simulink model "EE684_Project"  (R2023b)
settings: Solver=ode23t  StartTime=0.0  StopTime=1  RelTol=1e-3
undefined symbols (not defined in the file): acSupply, acSupplyController, bms, bmsController, boostController, connectedLoad, dcVoltage, Ion, Lithium, maxSoC, maxVdc, minIrrad, minSoC, minVdc, olTime, sensor, solarPanel, solarPlant
libraries: fl_lib x25, nesl_utility x23, ee_lib x12, spsSeriesRLCBranchLib x8, simulink x6, eePwmGenerator x4, spsIGBTDiodeLib x4, simulink_extras x2, spsCurrentMeasurementLib x2, spsMosfetLib x2, slpidlib x2, spsVoltageMeasurementLib x2
(part 2 of 2)

== system EE684_Project/AC System/AC Supply Controller ==
  note: Voltage Control
  note: Current control
  Modulating Signal : Subsystem
  Sine Wave1 : Sin  Amplitude=acSupply.supplyVoltage*1.414  Frequency=acSupply.frequency*2*pi  SampleTime=1/(30*2*pi*acSupply.frequency)
  Sum5 : Sum  Inputs=|+-
  Sum8 : Sum  Inputs=|+-
  Transfer Fcn1 : TransferFcn  Denominator=[1e-4 1]
  Voltage control2 : Subsystem
  d-axis current control2 : Subsystem
  act : Outport  VectorParamsAs1DForOutWhenUnconnected=off
  wires:
  Modulating Signal/1(m1) -> act/1
  d-axis current control2/1(u) -> Modulating Signal/1(Vmod)
  [Vo] -> Modulating Signal/2(Vdc)
  Sum8/1 -> Voltage control2/1(e)
  [Vs] -> Sum8/2
  [Iac] -> Sum5/2
  Sum5/1 -> d-axis current control2/1(e)
  Sine Wave1/1 -> Transfer Fcn1/1
  Voltage control2/1(u) -> Sum5/1
  Transfer Fcn1/1 -> Sum8/1

== system EE684_Project/AC System/Complex Load ==
  AC Voltage Sensor1 : Subsystem
      mask Display: disp('v')
  DC Current Sensor : Subsystem
      mask Display: disp('i')
  Inductor : ee_lib/Passive/Inductor  Commented=on  l=0 H  enable_L_tol=0  L_tol=5  tol_distribution=1  nSigma=4  r=0 Ohm  g=1e-9 1/Ohm  enable_operating_limits=0  operating_limit_action=2  max_working_current=1 A  power_rating=1 W  enable_faults=ee.enum.enable.no  fault_action=simscape.enum.assert.action.none  lambdaPercent=50  k_faulted=0.9999  turnsShort=0  openCct=0  groundShort=0  groundShortG=0 1/Ohm  tau_fault=1e-3 s  fault_trigger=ee.enum.faults.faultTrigger.temporal  t_fault=1 s  max_permissible_voltage=100 V  n_fail_on_voltage=1  max_permissible_current=1 A  t_fail_on_current=1 s  i_L_specify=off  i_L_priority=High  i_L=0 A  i_L_nominal_specify=off  i_L_nominal_unit=A  i_L_nominal_value=1
  Load Calculation : Subsystem
  Load Resistance : fl_lib/Electrical/Electrical Elements/Variable Resistor  Rmin=0 Ohm  thermalEnable=false  thermal_mass=1 J/K  i_specify=off  i_priority=None  i=5 A  i_nominal_specify=off  i_nominal_unit=A  i_nominal_value=1  v_specify=off  v_priority=None  v=0 V  v_nominal_specify=off  v_nominal_unit=V  v_nominal_value=1  T_specify=off  T_priority=None  T=300 K  T_nominal_specify=off  T_nominal_unit=K  T_nominal_value=1
  Variable Inductor : ee_lib/Passive/Variable Inductor  prm=1  Lmin=1e-6 H  g=1e-9 1/Ohm  i0=0 A  phi0=0 Wb
      settings: InternalSimscapePortConfiguration="{\"Bottom\":[],\"Left\":[{\"id\":\"L\",\"label\":\"L\",\"type\":\"input\"},{\"id\":\"p\",\"label\":\"+\",\"type\":\"foundation.electrical.electrical\"}],\"Right\":[{\"id\":\"n\",\"label\":\"-\",\"type\":\"foundation.electrical.electrical\"}],\"Top\":[]}"
  P : PMIOPort  Side=Left
  N : PMIOPort  Port=2  Side=Left
  connections:
  AC Voltage Sensor1/LConn1 -- N/RConn1 -- Variable Inductor/RConn1
  Load Resistance/LConn2 -- DC Current Sensor/LConn1
  DC Current Sensor/RConn1 -- P/RConn1 -- AC Voltage Sensor1/RConn1
  Variable Inductor/LConn2 -- Load Resistance/RConn1
  Load Calculation/RConn1 -- Load Resistance/LConn1
  Load Calculation/RConn2 -- Variable Inductor/LConn1

== system EE684_Project/AC System/Load Flag ==
  Data Type Conversion1 : DataTypeConversion  SaturateOnIntegerOverflow=off  RndMeth=Floor
  NOT : Logic  Operator=NOT  IconShape=distinctive  AllPortsSameDT=off  OutDataTypeStr=boolean
  OR : Logic  Operator=OR  IconShape=distinctive  AllPortsSameDT=off  OutDataTypeStr=boolean
  Simulink-PS Converter2 : nesl_utility/Simulink-PS Converter  PhysicalDomain=network_engine_domain  SubClassName=ps_input  LeftPortType=input  RightPortType=output  PseudoPeriodic=off  Frequencies=[]  NoiseDistribution=none  NoiseParameters=[]  Unit=1  AffineConversion=off  FilteringAndDerivatives=provide  SimscapeFilterOrder=1  InputFilterTimeConstant=0.001  UdotUserProvided=0
  CB : PMIOPort  Side=Right
  wires:
  [loadShutDown] -> OR/1
  Data Type Conversion1/1 -> Simulink-PS Converter2/1
  [ShutDown] -> OR/2  "System Status"
  OR/1 -> NOT/1
  NOT/1 -> Data Type Conversion1/1
  connections:
  Simulink-PS Converter2/RConn1 -- CB/RConn1

== system EE684_Project/AC System/Single Phase Inverter ==
  DC Current Sensor : Subsystem
      mask Display: disp('i')
  Power Circuit : Subsystem  Variant=on  VariantControl=Variant1
  + : PMIOPort  Side=Left
  P : PMIOPort  Port=2  Side=Right
  N : PMIOPort  Port=3  Side=Right
  - : PMIOPort  Port=4  Side=Left
  wires:
  [acMod] -> Power Circuit/1(m)
  [ShutDown] -> Power Circuit/2(TripSig)
  connections:
  +/RConn1 -- Power Circuit/LConn1
  -/RConn1 -- Power Circuit/LConn2
  P/RConn1 -- DC Current Sensor/LConn1
  N/RConn1 -- Power Circuit/RConn2
  DC Current Sensor/RConn1 -- Power Circuit/RConn1

== system EE684_Project/BMS/DC Battery Current Sensor1 ==
  Current Sensor : fl_lib/Electrical/Electrical Sensors/Current Sensor
  PS-Simulink Converter : nesl_utility/PS-Simulink Converter  PhysicalDomain=network_engine_domain  SubClassName=ps_output  LeftPortType=input  RightPortType=output  PseudoPeriodic=off  Frequencies=[]  VectorFormat=1-D array  Unit=1  AffineConversion=off
  Sensor dynamics : TransferFcn  Numerator=1  Denominator=[1/sensor.samplingFreq 1]
  - : PMIOPort  Side=Left
  + : PMIOPort  Port=2  Side=Right
  tag scope: Ibattery=global
  wires:
  PS-Simulink Converter/1 -> Sensor dynamics/1
  Sensor dynamics/1 -> [Ibattery]
  connections:
  Current Sensor/RConn1 -- PS-Simulink Converter/LConn1
  +/RConn1 -- Current Sensor/LConn1
  Current Sensor/RConn2 -- -/RConn1

== system EE684_Project/BMS/DC Battery Current Sensor2 ==
  Current Sensor : fl_lib/Electrical/Electrical Sensors/Current Sensor
  PS-Simulink Converter : nesl_utility/PS-Simulink Converter  PhysicalDomain=network_engine_domain  SubClassName=ps_output  LeftPortType=input  RightPortType=output  PseudoPeriodic=off  Frequencies=[]  VectorFormat=1-D array  Unit=1  AffineConversion=off
  Sensor dynamics : TransferFcn  Numerator=1  Denominator=[1/sensor.samplingFreq 1]
  - : PMIOPort  Side=Left
  + : PMIOPort  Port=2  Side=Right
  tag scope: Ibatval=global
  wires:
  PS-Simulink Converter/1 -> Sensor dynamics/1
  Sensor dynamics/1 -> [Ibatval]
  connections:
  Current Sensor/RConn1 -- PS-Simulink Converter/LConn1
  +/RConn1 -- Current Sensor/LConn1
  Current Sensor/RConn2 -- -/RConn1

== system EE684_Project/BMS/DC Battery Voltage Sensor ==
  PS-Simulink Converter : nesl_utility/PS-Simulink Converter  PhysicalDomain=network_engine_domain  SubClassName=ps_output  LeftPortType=input  RightPortType=output  PseudoPeriodic=off  Frequencies=[]  VectorFormat=1-D array  Unit=1  AffineConversion=off
  Sensor dynamics : TransferFcn  Numerator=1  Denominator=[1/sensor.samplingFreq 1]
  Voltage Sensor : fl_lib/Electrical/Electrical Sensors/Voltage Sensor
      settings: LogSimulationData=on
  - : PMIOPort  Side=Left
  + : PMIOPort  Port=2  Side=Right
  tag scope: Vbat=global
  wires:
  PS-Simulink Converter/1 -> Sensor dynamics/1
  Sensor dynamics/1 -> [Vbat]
  connections:
  Voltage Sensor/LConn1 -- +/RConn1
  Voltage Sensor/RConn1 -- PS-Simulink Converter/LConn1
  Voltage Sensor/RConn2 -- -/RConn1

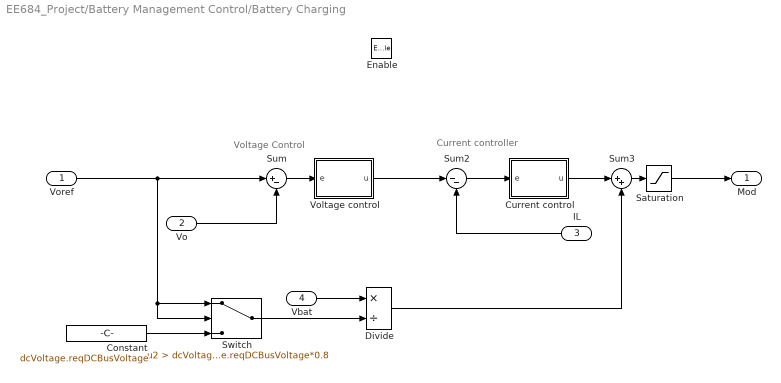
== system EE684_Project/Battery Management Control/Battery Charging ==
  note: Current controller
  note: Voltage Control
  Voref : Inport
  Vo : Inport  Port=2
  IL : Inport  Port=3
  Vbat : Inport  Port=4
  Enable : EnablePort  StatesWhenEnabling=reset
  Constant : Constant  Value=dcVoltage.reqDCBusVoltage
  Current control : Subsystem
  Divide : Product  Inputs=*/
  Saturation : Saturate  UpperLimit=1  LowerLimit=0
  Sum : Sum  Inputs=|+-
  Sum2 : Sum  Inputs=|--
  Sum3 : Sum  Inputs=|++
  Switch : Switch  Criteria=u2 > Threshold  Threshold=dcVoltage.reqDCBusVoltage*0.8  SaturateOnIntegerOverflow=off  InputSameDT=off
  Voltage control : Subsystem
  Mod : Outport
  wires:
  Voltage control/1(u) -> Sum2/1
  Voref/1 -> Switch/2, Switch/1, Sum/1
  Switch/1 -> Divide/2
  Sum2/1 -> Current control/1(e)
  Vo/1 -> Sum/2
  Current control/1(u) -> Sum3/1
  IL/1 -> Sum2/2
  Sum/1 -> Voltage control/1(e)
  Sum3/1 -> Saturation/1
  Saturation/1 -> Mod/1
  Constant/1 -> Switch/3
  Divide/1 -> Sum3/2
  Vbat/1 -> Divide/1

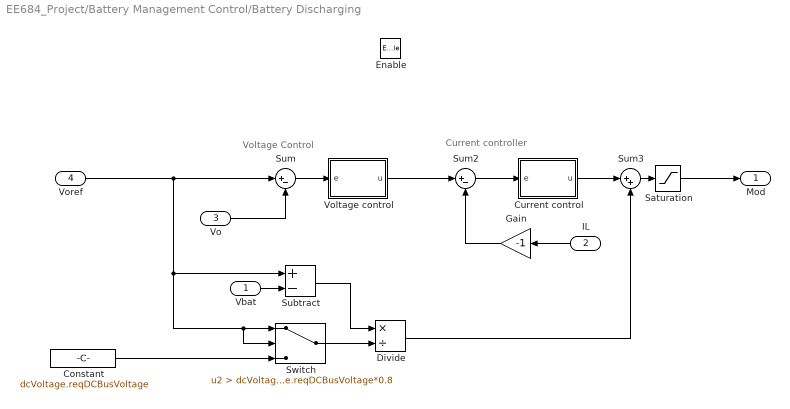
== system EE684_Project/Battery Management Control/Battery Discharging ==
  note: Current controller
  note: Voltage Control
  Vbat : Inport
  IL : Inport  Port=2
  Vo : Inport  Port=3
  Voref : Inport  Port=4
  Enable : EnablePort  StatesWhenEnabling=reset
  Constant : Constant  Value=dcVoltage.reqDCBusVoltage
  Current control : Subsystem
  Divide : Product  Inputs=*/
  Gain : Gain  Gain=-1
  Saturation : Saturate  UpperLimit=1  LowerLimit=0
  Subtract : Sum  Inputs=+-
  Sum : Sum  Inputs=|+-
  Sum2 : Sum  Inputs=|+-
  Sum3 : Sum  Inputs=|++
  Switch : Switch  Criteria=u2 > Threshold  Threshold=dcVoltage.reqDCBusVoltage*0.8  SaturateOnIntegerOverflow=off  InputSameDT=off
  Voltage control : Subsystem
  Mod : Outport
  wires:
  Voltage control/1(u) -> Sum2/1
  Voref/1 -> Sum/1, Subtract/1, Switch/2, Switch/1
  Switch/1 -> Divide/2
  Subtract/1 -> Divide/1
  Sum2/1 -> Current control/1(e)
  Vo/1 -> Sum/2
  Current control/1(u) -> Sum3/1
  IL/1 -> Gain/1
  Sum/1 -> Voltage control/1(e)
  Sum3/1 -> Saturation/1
  Saturation/1 -> Mod/1
  Vbat/1 -> Subtract/2
  Constant/1 -> Switch/3
  Gain/1 -> Sum2/2
  Divide/1 -> Sum3/2

== system EE684_Project/Battery Management Control/Charging ==
  mod : Inport
  Enable : EnablePort  StatesWhenEnabling=reset
  Constant : Constant  Value=0
  Gain : Gain
  Gain2 : Gain  Gain=5
  Rate Transition1 : RateTransition
  S1 : Outport
  S2 : Outport  Port=2
  wires:
  mod/1 -> Gain2/1
  Gain2/1 -> S1/1
  Gain/1 -> Rate Transition1/1
  Constant/1 -> Gain/1
  Rate Transition1/1 -> S2/1

== system EE684_Project/Battery Management Control/Discharging ==
  mod : Inport
  Enable : EnablePort  StatesWhenEnabling=reset
  Constant : Constant  Value=0
  Gain : Gain  Gain=5
  Gain1 : Gain
  Rate Transition1 : RateTransition
  S2 : Outport
  S1 : Outport  Port=2
  wires:
  mod/1 -> Gain/1
  Gain1/1 -> Rate Transition1/1
  Constant/1 -> Gain1/1
  Rate Transition1/1 -> S1/1
  Gain/1 -> S2/1

== system EE684_Project/Battery Management Control/Isolate ==
  Enable : EnablePort  StatesWhenEnabling=reset
  Constant : Constant  Value=0
  Constant1 : Constant  Value=0
  Gain : Gain
  Gain1 : Gain
  Rate Transition : RateTransition
  Rate Transition1 : RateTransition
  S2 : Outport
  S1 : Outport  Port=2
  wires:
  Constant/1 -> Gain/1
  Constant1/1 -> Gain1/1
  Gain/1 -> Rate Transition/1
  Gain1/1 -> Rate Transition1/1
  Rate Transition/1 -> S1/1
  Rate Transition1/1 -> S2/1

== system EE684_Project/Battery Management Control/PWM ==
  mod : Inport
  PWM Generator : eePwmGenerator/PWM Generator  CarrCount=Up  Tper=1/bms.batteryConverterSwitchingFrequency  Tdelay=0  Ts=1/(10*bms.batteryConverterSwitchingFrequency)
  Rate Transition1 : RateTransition  OutPortSampleTime=1/(10*bms.batteryConverterSwitchingFrequency)
  PWM : Outport
  wires:
  Rate Transition1/1 -> PWM Generator/1
  mod/1 -> Rate Transition1/1
  PWM Generator/1 -> PWM/1

== system EE684_Project/Boost Converter/AC Current Sensor1 ==
  Current Sensor : fl_lib/Electrical/Electrical Sensors/Current Sensor
  PS-Simulink Converter : nesl_utility/PS-Simulink Converter  PhysicalDomain=network_engine_domain  SubClassName=ps_output  LeftPortType=input  RightPortType=output  PseudoPeriodic=off  Frequencies=[]  VectorFormat=1-D array  Unit=1  AffineConversion=off
  Sensor dynamics : TransferFcn  Numerator=1  Denominator=[1/sensor.samplingFreq 1]
  - : PMIOPort  Side=Left
  + : PMIOPort  Port=2  Side=Right
  tag scope: IL=global
  wires:
  PS-Simulink Converter/1 -> Sensor dynamics/1
  Sensor dynamics/1 -> [IL]
  connections:
  Current Sensor/RConn1 -- PS-Simulink Converter/LConn1
  +/RConn1 -- Current Sensor/LConn1
  Current Sensor/RConn2 -- -/RConn1

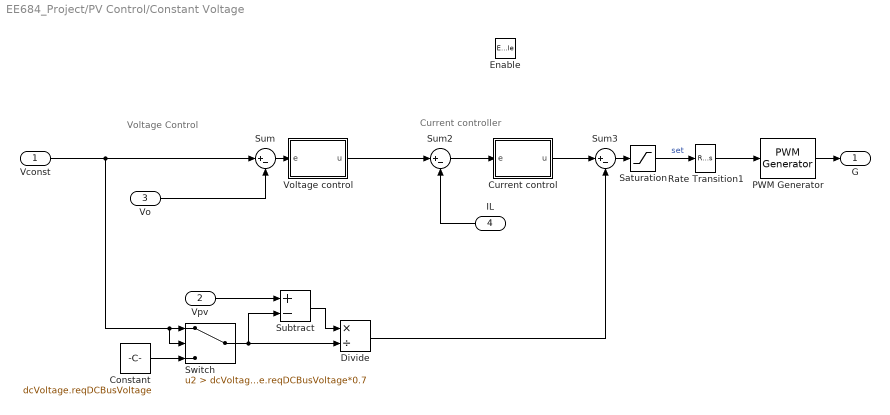
== system EE684_Project/PV Control/Constant Voltage ==
  note: Current controller
  note: Voltage Control
  Vconst : Inport
  Vpv : Inport  Port=2
  "Vo " : Inport  Port=3
  IL : Inport  Port=4
  Enable : EnablePort  StatesWhenEnabling=reset
  Constant : Constant  Value=dcVoltage.reqDCBusVoltage
  Current control : Subsystem
  Divide : Product  Inputs=*/
  PWM Generator : eePwmGenerator/PWM Generator  CarrCount=Up  Tper=1/solarPlant.converterSwitchingFrequency  Tdelay=0  Ts=1/(10*solarPlant.converterSwitchingFrequency)
  Rate Transition1 : RateTransition  OutPortSampleTime=1/(10*solarPlant.converterSwitchingFrequency)
  Saturation : Saturate  UpperLimit=1  LowerLimit=0
  Subtract : Sum  Inputs=+-
  Sum : Sum  Inputs=|+-
  Sum2 : Sum  Inputs=|+-
  Sum3 : Sum  Inputs=|+-
  Switch : Switch  Criteria=u2 > Threshold  Threshold=dcVoltage.reqDCBusVoltage*0.7  SaturateOnIntegerOverflow=off  InputSameDT=off
  Voltage control : Subsystem
  G : Outport
  wires:
  Switch/1 -> Divide/2, Subtract/2
  Constant/1 -> Switch/3
  "Vo "/1 -> Sum/2
  Vconst/1 -> Switch/2, Switch/1, Sum/1
  Divide/1 -> Sum3/2
  PWM Generator/1 -> G/1
  Rate Transition1/1 -> PWM Generator/1
  Sum3/1 -> Saturation/1
  Vpv/1 -> Subtract/1
  Sum/1 -> Voltage control/1(e)
  Voltage control/1(u) -> Sum2/1
  Current control/1(u) -> Sum3/1
  Sum2/1 -> Current control/1(e)
  Subtract/1 -> Divide/1
  Saturation/1 -> Rate Transition1/1  "set"
  IL/1 -> Sum2/2

== system EE684_Project/PV Control/Maximum Power Point ==
  "IL " : Inport
  "Vo " : Inport  Port=2
  Vpv : Inport  Port=3
  Ipv : Inport  Port=4
  Enable : EnablePort  StatesWhenEnabling=reset
  MPPT : Subsystem
  MPPT Subsystem : Subsystem  TreatAsAtomicUnit=on
  Rate Transition : RateTransition  OutPortSampleTime=0.02
  ZOH/4 : ZeroOrderHold  SampleTime=solarPlant.timeMPPT
  Gmpp : Outport
  Vmpp : Outport  Port=2
  wires:
  ZOH/4/1 -> MPPT/2(Vpv)
  Rate Transition/1 -> MPPT/1(Ipv)
  MPPT/1(Vmpp) -> Vmpp/1, MPPT Subsystem/1(VpvRef)
  "Vo "/1 -> MPPT Subsystem/4("Vo ")
  Ipv/1 -> Rate Transition/1
  Vpv/1 -> MPPT Subsystem/2(Vpv), ZOH/4/1
  MPPT Subsystem/1(G) -> Gmpp/1
  "IL "/1 -> MPPT Subsystem/3(IL)

== system EE684_Project/PV Control/PV Isolate ==
  Enable : EnablePort  StatesWhenEnabling=reset
  Constant : Constant  Value=0
  Gain : Gain
  Rate Transition : RateTransition
  Gmpp : Outport
  wires:
  Constant/1 -> Gain/1
  Gain/1 -> Rate Transition/1
  Rate Transition/1 -> Gmpp/1

== system EE684_Project/Solar Plant/Load Flag ==
  Data Type Conversion1 : DataTypeConversion  SaturateOnIntegerOverflow=off  RndMeth=Floor
  NOT : Logic  Operator=NOT  IconShape=distinctive  AllPortsSameDT=off  OutDataTypeStr=boolean
  Simulink-PS Converter2 : nesl_utility/Simulink-PS Converter  PhysicalDomain=network_engine_domain  SubClassName=ps_input  LeftPortType=input  RightPortType=output  PseudoPeriodic=off  Frequencies=[]  NoiseDistribution=none  NoiseParameters=[]  Unit=1  AffineConversion=off  FilteringAndDerivatives=provide  SimscapeFilterOrder=1  InputFilterTimeConstant=0.001  UdotUserProvided=0
  CB : PMIOPort  Side=Right
  wires:
  Data Type Conversion1/1 -> Simulink-PS Converter2/1
  [ShutDown] -> NOT/1
  NOT/1 -> Data Type Conversion1/1
  connections:
  Simulink-PS Converter2/RConn1 -- CB/RConn1

== system EE684_Project/Solar Plant/Solar Panel ==
  Current-Controlled Current Source : fl_lib/Electrical/Electrical Sources/Current-Controlled Current Source  K=-1*(solarPanel.numParallelCell-1)  i1_specify=off  i1_priority=None  i1=0 A  i1_nominal_specify=off  i1_nominal_unit=A  i1_nominal_value=1  i2_specify=off  i2_priority=None  i2=0 A  i2_nominal_specify=off  i2_nominal_unit=A  i2_nominal_value=1
      settings: InternalSimscapePortConfiguration="{\"Bottom\":[],\"Left\":[{\"id\":\"p1\",\"label\":\"+\",\"type\":\"foundation.electrical.electrical\"},{\"id\":\"head\",\"label\":\"\",\"type\":\"foundation.electrical.electrical\"}],\"Right\":[{\"id\":\"n1\",\"label\":\"-\",\"type\":\"foundation.electrical.electrical\"},{\"id\":\"tail\",\"label\":\"\",\"type\":\"foundation.electrical.electrical\"}],\"Top\":[]}"
  Solar Cell : ee_lib/Sources/Solar Cell  prm=1  Isc=solarPanel.shortCircuitCurrentPV/solarPanel.numParallelCell A  Voc=solarPanel.openCircuitVoltagePV/solarPanel.numSeriesCell V  Is=1e-6 A  Is2=0 A  Iph=7.34 A  Ir0=solarPanel.irradianceMeasurement W/m^2  ec=solarPanel.qualityFactor  N2=2  Rs=solarPanel.seriesResistance Ohm  Rp=inf Ohm  N_series=solarPanel.numSeriesCell-1  N_parallel=1  TIPH1=solarPanel.currentTemperatureCoeff 1/K  EG=1.11 eV  TXIS1=solarPanel.temperatureExponent  TXIS2=3  TRS1=0  TRP1=0  Tmeas=solarPanel.temperatureMeasurement degC  TFIXED=environment.temperature degC  thermal_mass=100 J/K  initial_temperature=25 degC
  Ir : PMIOPort  Side=Left
  + : PMIOPort  Port=2  Side=Right
  - : PMIOPort  Port=3  Side=Right
  connections:
  Current-Controlled Current Source/LConn2 -- -/RConn1 -- Solar Cell/RConn1
  Ir/RConn1 -- Solar Cell/LConn1
  Current-Controlled Current Source/LConn1 -- Solar Cell/LConn2
  Current-Controlled Current Source/RConn1 -- Current-Controlled Current Source/RConn2 -- +/RConn1

== system EE684_Project/AC System/AC Supply Controller/Modulating Signal ==
  Vmod : Inport
  Vdc : Inport  Port=2
  Normalize by DC voltage and disable if DC volts too low : Subsystem
  "[-1,1]" : Saturate  UpperLimit=1  LowerLimit=-1
  m1 : Outport  VectorParamsAs1DForOutWhenUnconnected=off
  wires:
  Normalize by DC voltage and disable if DC volts too low/1(y) -> "[-1,1]"/1
  Vdc/1 -> Normalize by DC voltage and disable if DC volts too low/2(v_dc)
  Vmod/1 -> Normalize by DC voltage and disable if DC volts too low/1(u)
  "[-1,1]"/1 -> m1/1

== system EE684_Project/AC System/AC Supply Controller/Voltage control2 ==
  e : Inport
  Integrator : Integrator  LimitOutput=on  UpperSaturationLimit=acSupply.maxPowerACCurrent*sqrt(2)*1.1  LowerSaturationLimit=-acSupply.maxPowerACCurrent*sqrt(2)*1.1
  Ki : Gain  Gain=1/(acSupplyController.voltagePole)
  Kp : Gain  Gain=acSupplyController.voltageGain
  Saturation : Saturate  UpperLimit=acSupply.maxPowerACCurrent*sqrt(2)*10  LowerLimit=-1*acSupply.maxPowerACCurrent*sqrt(2)*10
  Scope : Scope
  Sum7 : Sum  Inputs=|++
  u : Outport  VectorParamsAs1DForOutWhenUnconnected=off
  wires:
  Integrator/1 -> Sum7/2
  Saturation/1 -> Scope/1, u/1
  Sum7/1 -> Saturation/1
  e/1 -> Kp/1
  Kp/1 -> Ki/1, Sum7/1
  Ki/1 -> Integrator/1

== system EE684_Project/AC System/AC Supply Controller/d-axis current control2 ==
  e : Inport
  Integrator : Integrator  LimitOutput=on  UpperSaturationLimit=acSupplyController.currentVoltMax  LowerSaturationLimit=-acSupplyController.currentVoltMax
  Ki : Gain  Gain=1/acSupplyController.currentPole
  Kp : Gain  Gain=acSupplyController.currentGain
  Saturation : Saturate  UpperLimit=acSupplyController.currentVoltMax  LowerLimit=-1*acSupplyController.currentVoltMax
  Scope : Scope
  Sum7 : Sum  Inputs=|++
  u : Outport  VectorParamsAs1DForOutWhenUnconnected=off
  wires:
  Integrator/1 -> Sum7/2
  Saturation/1 -> Scope/1, u/1
  Sum7/1 -> Saturation/1
  e/1 -> Kp/1
  Kp/1 -> Ki/1, Sum7/1
  Ki/1 -> Integrator/1

== system EE684_Project/AC System/Complex Load/AC Voltage Sensor1 ==
  PS-Simulink Converter : nesl_utility/PS-Simulink Converter  PhysicalDomain=network_engine_domain  SubClassName=ps_output  LeftPortType=input  RightPortType=output  PseudoPeriodic=off  Frequencies=[]  VectorFormat=1-D array  Unit=1  AffineConversion=off
  Sensor dynamics : TransferFcn  Numerator=1  Denominator=[1/sensor.samplingFreq 1]
  Voltage Sensor : fl_lib/Electrical/Electrical Sensors/Voltage Sensor
  - : PMIOPort  Side=Left
  + : PMIOPort  Port=2  Side=Right
  tag scope: Vs=global
  wires:
  PS-Simulink Converter/1 -> Sensor dynamics/1
  Sensor dynamics/1 -> [Vs]
  connections:
  Voltage Sensor/RConn2 -- -/RConn1
  Voltage Sensor/RConn1 -- PS-Simulink Converter/LConn1
  Voltage Sensor/LConn1 -- +/RConn1

== system EE684_Project/AC System/Complex Load/DC Current Sensor ==
  Current Sensor : fl_lib/Electrical/Electrical Sensors/Current Sensor
      settings: LogSimulationData=on
  PS-Simulink Converter : nesl_utility/PS-Simulink Converter  PhysicalDomain=network_engine_domain  SubClassName=ps_output  LeftPortType=input  RightPortType=output  PseudoPeriodic=off  Frequencies=[]  VectorFormat=1-D array  Unit=1  AffineConversion=off
  Sensor dynamics : TransferFcn  Numerator=1  Denominator=[1/sensor.samplingFreq 1]
  - : PMIOPort  Side=Left
  + : PMIOPort  Port=2  Side=Right
  tag scope: Iload=global
  wires:
  PS-Simulink Converter/1 -> Sensor dynamics/1
  Sensor dynamics/1 -> [Iload]
  connections:
  Current Sensor/RConn2 -- -/RConn1
  +/RConn1 -- Current Sensor/LConn1
  Current Sensor/RConn1 -- PS-Simulink Converter/LConn1

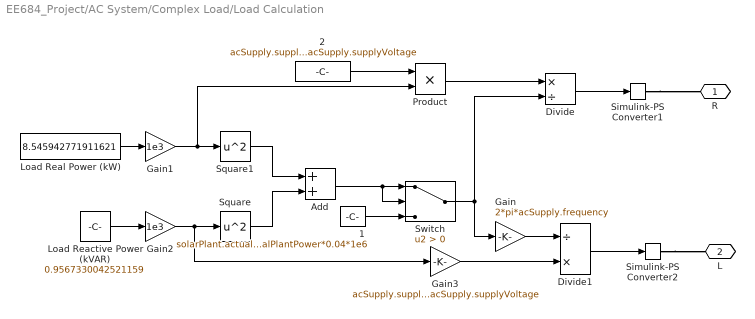
== system EE684_Project/AC System/Complex Load/Load Calculation ==
  " 1" : Constant  Value=solarPlant.actualPlantPower*solarPlant.actualPlantPower*0.04*1e6
  " 2" : Constant  Value=acSupply.supplyVoltage*acSupply.supplyVoltage
  " Load Reactive Power (kVAR)" : Constant  Value=0.9567330042521159
  " Load Real Power (kW)" : Constant  Value=8.545942771911621
  Add : Sum
  Divide : Product  Inputs=*/
  Divide1 : Product  Inputs=/*
  Gain : Gain  Gain=2*pi*acSupply.frequency
  Gain1 : Gain  Gain=1e3
  Gain2 : Gain  Gain=1e3
  Gain3 : Gain  Gain=acSupply.supplyVoltage*acSupply.supplyVoltage
  Product : Product
  Simulink-PS Converter1 : nesl_utility/Simulink-PS Converter  PhysicalDomain=network_engine_domain  SubClassName=ps_input  LeftPortType=input  RightPortType=output  PseudoPeriodic=off  Frequencies=[]  NoiseDistribution=none  NoiseParameters=[]  Unit=1  AffineConversion=off  FilteringAndDerivatives=provide  SimscapeFilterOrder=1  InputFilterTimeConstant=0.001  UdotUserProvided=0
  Simulink-PS Converter2 : nesl_utility/Simulink-PS Converter  PhysicalDomain=network_engine_domain  SubClassName=ps_input  LeftPortType=input  RightPortType=output  PseudoPeriodic=off  Frequencies=[]  NoiseDistribution=none  NoiseParameters=[]  Unit=1  AffineConversion=off  FilteringAndDerivatives=provide  SimscapeFilterOrder=1  InputFilterTimeConstant=0.001  UdotUserProvided=0
  Square : Math  Operator=square
  Square1 : Math  Operator=square
  Switch : Switch  Criteria=u2 > Threshold  SaturateOnIntegerOverflow=off  InputSameDT=off
  R : PMIOPort  Side=Right
  L : PMIOPort  Port=2  Side=Right
  wires:
  " Load Real Power (kW)"/1 -> Gain1/1
  " 1"/1 -> Switch/3
  Divide/1 -> Simulink-PS Converter1/1
  " Load Reactive Power (kVAR)"/1 -> Gain2/1
  Square1/1 -> Add/1
  Square/1 -> Add/2
  Add/1 -> Switch/2, Switch/1
  " 2"/1 -> Product/1
  Product/1 -> Divide/1
  Switch/1 -> Divide/2, Gain/1
  Gain/1 -> Divide1/1
  Divide1/1 -> Simulink-PS Converter2/1
  Gain1/1 -> Product/2, Square1/1
  Gain2/1 -> Square/1, Gain3/1
  Gain3/1 -> Divide1/2
  connections:
  Simulink-PS Converter1/RConn1 -- R/RConn1
  Simulink-PS Converter2/RConn1 -- L/RConn1

== system EE684_Project/AC System/Single Phase Inverter/DC Current Sensor ==
  Current Sensor : fl_lib/Electrical/Electrical Sensors/Current Sensor
      settings: LogSimulationData=on
  PS-Simulink Converter : nesl_utility/PS-Simulink Converter  PhysicalDomain=network_engine_domain  SubClassName=ps_output  LeftPortType=input  RightPortType=output  PseudoPeriodic=off  Frequencies=[]  VectorFormat=1-D array  Unit=1  AffineConversion=off
  Sensor dynamics : TransferFcn  Numerator=1  Denominator=[1/sensor.samplingFreq 1]
  - : PMIOPort  Side=Left
  + : PMIOPort  Port=2  Side=Right
  tag scope: Iac=global
  wires:
  PS-Simulink Converter/1 -> Sensor dynamics/1
  Sensor dynamics/1 -> [Iac]
  connections:
  Current Sensor/RConn2 -- -/RConn1
  +/RConn1 -- Current Sensor/LConn1
  Current Sensor/RConn1 -- PS-Simulink Converter/LConn1

== system EE684_Project/AC System/Single Phase Inverter/Power Circuit ==
  m : Inport
  TripSig : Inport  Port=2
  Average : Subsystem  VariantControl=average
  Discrete : Subsystem  VariantControl=discrete
  P : PMIOPort  Side=Right
  + : PMIOPort  Port=2  Side=Left
  - : PMIOPort  Port=3  Side=Left
  N : PMIOPort  Port=4  Side=Right

== system EE684_Project/Battery Management Control/Battery Charging/Current control ==
  e : Inport
  1/T : Gain  Gain=1/bms.chargeCurrentZeroTimeConst
  Integrator : Integrator  LimitOutput=on  UpperSaturationLimit=1.3  LowerSaturationLimit=-1.3
  Kp : Gain  Gain=bms.chargeCurrentGain
  Saturation : Saturate  UpperLimit=1.5  LowerLimit=-1.5
  Sum7 : Sum  Inputs=|++
  u : Outport  VectorParamsAs1DForOutWhenUnconnected=off
  wires:
  Integrator/1 -> Sum7/2
  Saturation/1 -> u/1
  Sum7/1 -> Saturation/1
  e/1 -> Kp/1
  Kp/1 -> 1/T/1, Sum7/1
  1/T/1 -> Integrator/1

== system EE684_Project/Battery Management Control/Battery Charging/Voltage control ==
  e : Inport
  1/T : Gain  Gain=1/bmsController.chosenChargeVoltageZeroTimeConst
  Integrator : Integrator  LimitOutput=on  UpperSaturationLimit=bms.maximumChargingCurrentLimit  LowerSaturationLimit=-1*bms.maximumChargingCurrentLimit
  Kp : Gain  Gain=bmsController.chosenChargeVoltageGain
  Saturation : Saturate  UpperLimit=bms.maximumChargingCurrentLimit  LowerLimit=-1*bms.maximumChargingCurrentLimit
  Sum7 : Sum  Inputs=|++
  u : Outport  VectorParamsAs1DForOutWhenUnconnected=off
  wires:
  Integrator/1 -> Sum7/2
  Saturation/1 -> u/1
  e/1 -> Kp/1
  Kp/1 -> 1/T/1, Sum7/1
  1/T/1 -> Integrator/1
  Sum7/1 -> Saturation/1

== system EE684_Project/Battery Management Control/Battery Discharging/Current control ==
  e : Inport
  1/T : Gain  Gain=1/bms.dischargeCurrentZeroTimeConst
  Integrator : Integrator  InitialCondition=1  LimitOutput=on  UpperSaturationLimit=1  LowerSaturationLimit=-0.5
  Kp : Gain  Gain=bms.dischargeCurrentGain
  Saturation : Saturate  UpperLimit=1  LowerLimit=-1
  Sum7 : Sum  Inputs=|++
  u : Outport  VectorParamsAs1DForOutWhenUnconnected=off
  wires:
  Integrator/1 -> Sum7/2
  Saturation/1 -> u/1
  Sum7/1 -> Saturation/1
  e/1 -> Kp/1
  Kp/1 -> 1/T/1, Sum7/1
  1/T/1 -> Integrator/1

== system EE684_Project/Battery Management Control/Battery Discharging/Voltage control ==
  e : Inport
  1/T : Gain  Gain=1/bmsController.chosenDischargeVoltageZeroTimeConst
  Integrator : Integrator  LimitOutput=on  UpperSaturationLimit=bms.maximumDisChargingCurrent  LowerSaturationLimit=-1*bms.maximumDisChargingCurrent
  Kp : Gain  Gain=bmsController.chosenDischargeVoltageGain
  Saturation : Saturate  UpperLimit=bms.maximumDisChargingCurrent  LowerLimit=-1*bms.maximumDisChargingCurrent
  Sum7 : Sum  Inputs=|++
  u : Outport  VectorParamsAs1DForOutWhenUnconnected=off
  wires:
  Integrator/1 -> Sum7/2
  Saturation/1 -> u/1
  e/1 -> Kp/1
  Kp/1 -> 1/T/1, Sum7/1
  1/T/1 -> Integrator/1
  Sum7/1 -> Saturation/1

== system EE684_Project/PV Control/Constant Voltage/Current control ==
  e : Inport
  Integrator : Integrator  LimitOutput=on  UpperSaturationLimit=1.5  LowerSaturationLimit=-1.5
  Ki : Gain  Gain=1/boostController.mppCurrentZeroTimeConst
  Kp : Gain  Gain=boostController.mppCurrentGain
  Saturation : Saturate  UpperLimit=1.5  LowerLimit=-1.5
  Sum7 : Sum  Inputs=|++
  u : Outport  VectorParamsAs1DForOutWhenUnconnected=off
  wires:
  Integrator/1 -> Sum7/2
  Saturation/1 -> u/1
  Sum7/1 -> Saturation/1
  e/1 -> Kp/1
  Kp/1 -> Ki/1, Sum7/1
  Ki/1 -> Integrator/1

== system EE684_Project/PV Control/Constant Voltage/Voltage control ==
  e : Inport
  1/T : Gain  Gain=1/boostController.mppVoltageZeroTimeConst
  Integrator : Integrator  LimitOutput=on  UpperSaturationLimit=boostController.mppVoltageLoopMax  LowerSaturationLimit=boostController.mppVoltageLoopMin
  Kp : Gain  Gain=boostController.mppVoltageGain
  Saturation : Saturate  UpperLimit=boostController.mppVoltageLoopMax  LowerLimit=boostController.mppVoltageLoopMin
  Sum7 : Sum  Inputs=|++
  u : Outport  VectorParamsAs1DForOutWhenUnconnected=off
  wires:
  Integrator/1 -> Sum7/2
  Saturation/1 -> u/1
  Sum7/1 -> Saturation/1
  e/1 -> Kp/1
  Kp/1 -> 1/T/1, Sum7/1
  1/T/1 -> Integrator/1

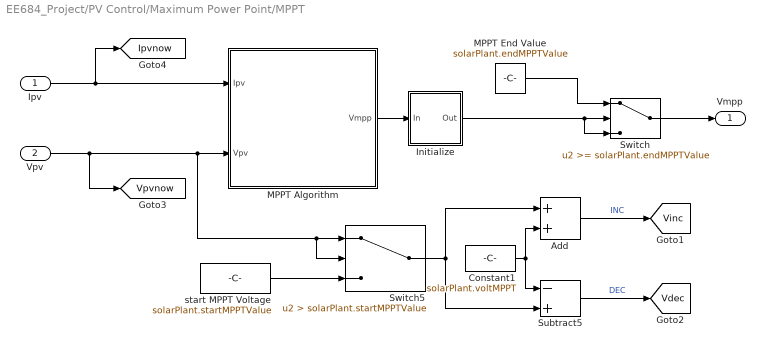
== system EE684_Project/PV Control/Maximum Power Point/MPPT ==
  Ipv : Inport
  Vpv : Inport  Port=2
  Add : Sum
  Constant1 : Constant  Value=solarPlant.voltMPPT
  Initialize : Subsystem
  MPPT Algorithm : Subsystem  Variant=on
  MPPT End Value : Constant  Value=solarPlant.endMPPTValue
  Subtract5 : Sum  Inputs=-+
  Switch : Switch  Threshold=solarPlant.endMPPTValue  SaturateOnIntegerOverflow=off  InputSameDT=off
  Switch5 : Switch  Criteria=u2 > Threshold  Threshold=solarPlant.startMPPTValue  SaturateOnIntegerOverflow=off  InputSameDT=off
  start MPPT Voltage : Constant  Value=solarPlant.startMPPTValue
  Vmpp : Outport  VectorParamsAs1DForOutWhenUnconnected=off
  tag scope: Ipvnow=global, Vdec=global, Vinc=global, Vpvnow=global
  wires:
  Switch5/1 -> Add/1, Subtract5/2
  Add/1 -> [Vinc]  "INC"
  start MPPT Voltage/1 -> Switch5/3
  Vpv/1 -> [Vpvnow], Switch5/2, Switch5/1, MPPT Algorithm/2(Vpv)
  Constant1/1 -> Add/2, Subtract5/1
  Subtract5/1 -> [Vdec]  "DEC"
  Ipv/1 -> [Ipvnow], MPPT Algorithm/1(Ipv)
  MPPT Algorithm/1(Vmpp) -> Initialize/1(In)
  Initialize/1(Out) -> Switch/3, Switch/2
  Switch/1 -> Vmpp/1
  MPPT End Value/1 -> Switch/1

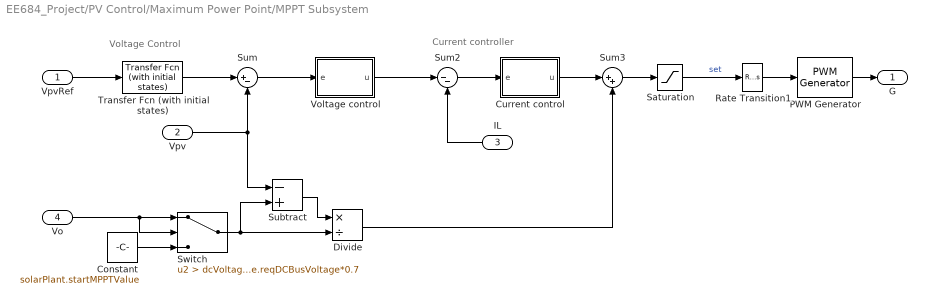
== system EE684_Project/PV Control/Maximum Power Point/MPPT Subsystem ==
  note: Current controller
  note: Voltage Control
  VpvRef : Inport
  Vpv : Inport  Port=2
  IL : Inport  Port=3
  "Vo " : Inport  Port=4
  Constant : Constant  Value=solarPlant.startMPPTValue
  Current control : Subsystem
  Divide : Product  Inputs=*/
  PWM Generator : eePwmGenerator/PWM Generator  CarrCount=Up  Tper=1/solarPlant.converterSwitchingFrequency  Tdelay=0  Ts=1/(10*solarPlant.converterSwitchingFrequency)
  Rate Transition1 : RateTransition  OutPortSampleTime=1/(10*solarPlant.converterSwitchingFrequency)
  Saturation : Saturate  UpperLimit=1  LowerLimit=0
  Subtract : Sum  Inputs=-+
  Sum : Sum  Inputs=|+-
  Sum2 : Sum  Inputs=|--
  Sum3 : Sum  Inputs=|++
  Switch : Switch  Criteria=u2 > Threshold  Threshold=dcVoltage.reqDCBusVoltage*0.7  SaturateOnIntegerOverflow=off  InputSameDT=off
  Transfer Fcn (with initial states) : simulink_extras/Additional Linear/Transfer Fcn (with initial states)  N=[1]  D=[0.00001 1]  X0=solarPlant.startMPPTValue
  Voltage control : Subsystem
  G : Outport
  wires:
  Subtract/1 -> Divide/1
  Voltage control/1(u) -> Sum2/1
  Current control/1(u) -> Sum3/1
  Sum2/1 -> Current control/1(e)
  "Vo "/1 -> Switch/2, Switch/1
  VpvRef/1 -> Transfer Fcn (with initial states)/1
  Constant/1 -> Switch/3
  Switch/1 -> Divide/2, Subtract/2
  Vpv/1 -> Subtract/1, Sum/2
  Saturation/1 -> Rate Transition1/1  "set"
  Rate Transition1/1 -> PWM Generator/1
  PWM Generator/1 -> G/1
  Divide/1 -> Sum3/2
  Sum/1 -> Voltage control/1(e)
  IL/1 -> Sum2/2
  Transfer Fcn (with initial states)/1 -> Sum/1
  Sum3/1 -> Saturation/1

== system EE684_Project/AC System/AC Supply Controller/Modulating Signal/Normalize by DC voltage and disable if DC volts too low ==
  u : Inport
  v_dc : Inport  Port=2
  Min DC voltage : Constant  Value=0.5*solarPlant.startMPPTValue
  Product1 : Product  Inputs=*/  InputSameDT=on  SaturateOnIntegerOverflow=on  OutDataTypeStr=Inherit: Same as first input
  Switch1 : Switch  Threshold=0.5*solarPlant.maxPowerVoltage  SaturateOnIntegerOverflow=off
  y : Outport  VectorParamsAs1DForOutWhenUnconnected=off
  wires:
  Min DC voltage/1 -> Switch1/3
  Switch1/1 -> Product1/2
  v_dc/1 -> Switch1/2, Switch1/1
  u/1 -> Product1/1
  Product1/1 -> y/1

== system EE684_Project/AC System/Single Phase Inverter/Power Circuit/Average ==
  m : Inport
  TripSig : Inport  Port=2
  Average-Value Chopper : ee_lib/Semiconductors & Converters/Converters/Average-Value Chopper  chopper_type=5  efficiency_option=1  efficiency_fixed=100  i_vec=[0, 2, 5] A  efficiency_vec=[90, 95, 98]
      settings: InternalSimscapePortConfiguration="{\"Bottom\":[],\"Left\":[{\"id\":\"DutyCycle\",\"label\":\"DutyCycle\",\"type\":\"input\"},{\"id\":\"p1\",\"label\":\"1+\",\"type\":\"foundation.electrical.electrical\"},{\"id\":\"n1\",\"label\":\"1-\",\"type\":\"foundation.electrical.electrical\"}],\"Right\":[{\"id\":\"p2\",\"label\":\"2+\",\"type\":\"foundation.electrical.electrical\"},{\"id\":\"n2\",\"label\":\"2-\",\"type\":\"foundation.electrical.electrical\"}],\"Top\":[]}"
  Map [-1,1] to [0,1] : Subsystem
  Simulink-PS Converter2 : nesl_utility/Simulink-PS Converter  PhysicalDomain=network_engine_domain  SubClassName=ps_input  LeftPortType=input  RightPortType=output  PseudoPeriodic=off  Frequencies=[]  NoiseDistribution=none  NoiseParameters=[]  Unit=1  AffineConversion=off  FilteringAndDerivatives=provide  SimscapeFilterOrder=1  InputFilterTimeConstant=0.001  UdotUserProvided=0
  Terminator : Terminator
  P : PMIOPort  Side=Right
  + : PMIOPort  Port=2  Side=Left
  - : PMIOPort  Port=3  Side=Left
  N : PMIOPort  Port=4  Side=Right
  wires:
  m/1 -> Simulink-PS Converter2/1
  TripSig/1 -> Terminator/1
  connections:
  Simulink-PS Converter2/RConn1 -- Map [-1,1] to [0,1]/LConn1
  Map [-1,1] to [0,1]/RConn1 -- Average-Value Chopper/LConn1
  N/RConn1 -- Average-Value Chopper/RConn2
  Average-Value Chopper/LConn3 -- -/RConn1
  +/RConn1 -- Average-Value Chopper/LConn2
  Average-Value Chopper/RConn1 -- P/RConn1

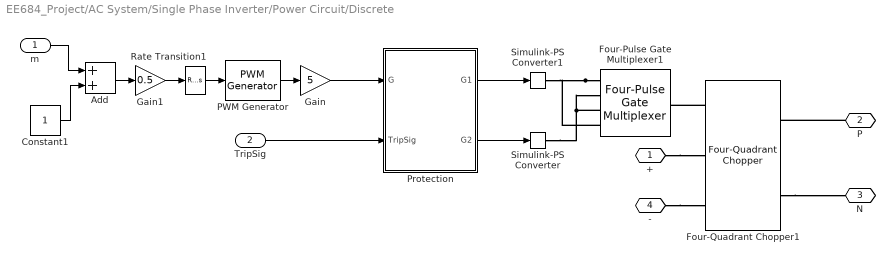
== system EE684_Project/AC System/Single Phase Inverter/Power Circuit/Discrete ==
  m : Inport
  TripSig : Inport  Port=2
  Add : Sum
  Constant1 : Constant
  Four-Pulse Gate Multiplexer1 : ee_lib/Semiconductors & Converters/Converters/Four-Pulse Gate Multiplexer  port_option=ee.enum.controlport.ps
      settings: InternalSimscapePortConfiguration="{\"Bottom\":[],\"Left\":[{\"id\":\"G1_ps\",\"label\":\"G1\",\"type\":\"input\"},{\"id\":\"G2_ps\",\"label\":\"G2\",\"type\":\"input\"},{\"id\":\"G3_ps\",\"label\":\"G3\",\"type\":\"input\"},{\"id\":\"G4_ps\",\"label\":\"G4\",\"type\":\"input\"}],\"Right\":[{\"id\":\"p\",\"label\":\"G\",\"type\":\"foundation.electrical.eight_phase\"}],\"Top\":[]}"
  Four-Quadrant Chopper1 : ee_lib/Semiconductors & Converters/Converters/Four-Quadrant Chopper  device_type=2  Vf=0.8 V  Ron=0.001 Ohm  Rds=0.001 Ohm  Goff=1e-5 1/Ohm  Vgt=1 V  Vgt_off=-1 V  Ih=1 A  Vth=2.5 V  K=0  diode_param=2  diode_Vf=0.8 V  diode_Ron=0.001 Ohm  diode_Goff=1e-5 1/Ohm  diode_C=50 nF  diode_iRM=-235 A  diode_iF=300 A  diode_idot=-50 A/us  diode_trr_param=1  diode_trr_factor=3  diode_trr=15 us  diode_Qrr=1500 s*uA  snubber_type=0  Cs=1e-7 F  Rs=0.1 Ohm
      settings: InternalSimscapePortConfiguration="{\"Bottom\":[],\"Left\":[{\"id\":\"G\",\"label\":\"G\",\"type\":\"foundation.electrical.eight_phase\"},{\"id\":\"p1\",\"label\":\"1+\",\"type\":\"foundation.electrical.electrical\"},{\"id\":\"n1\",\"label\":\"1-\",\"type\":\"foundation.electrical.electrical\"}],\"Right\":[{\"id\":\"p2\",\"label\":\"2+\",\"type\":\"foundation.electrical.electrical\"},{\"id\":\"n2\",\"label\":\"2-\",\"type\":\"foundation.electrical.electrical\"}],\"Top\":[]}"
  Gain : Gain  Gain=5
  Gain1 : Gain  Gain=0.5
  PWM Generator : eePwmGenerator/PWM Generator  CarrCount=Up  Tper=1/acSupply.inverterSwitchingFrequency  Tdelay=0  Ts=1/(10*acSupply.inverterSwitchingFrequency)
  Protection : Subsystem
  Rate Transition1 : RateTransition  OutPortSampleTime=1/(10*acSupply.inverterSwitchingFrequency)
  Simulink-PS Converter : nesl_utility/Simulink-PS Converter  PhysicalDomain=network_engine_domain  SubClassName=ps_input  LeftPortType=input  RightPortType=output  PseudoPeriodic=off  Frequencies=[]  NoiseDistribution=none  NoiseParameters=[]  Unit=1  AffineConversion=off  FilteringAndDerivatives=provide  SimscapeFilterOrder=1  InputFilterTimeConstant=0.001  UdotUserProvided=0
  Simulink-PS Converter1 : nesl_utility/Simulink-PS Converter  PhysicalDomain=network_engine_domain  SubClassName=ps_input  LeftPortType=input  RightPortType=output  PseudoPeriodic=off  Frequencies=[]  NoiseDistribution=none  NoiseParameters=[]  Unit=1  AffineConversion=off  FilteringAndDerivatives=provide  SimscapeFilterOrder=1  InputFilterTimeConstant=0.001  UdotUserProvided=0
  + : PMIOPort  Side=Left
  P : PMIOPort  Port=2  Side=Right
  N : PMIOPort  Port=3  Side=Right
  - : PMIOPort  Port=4  Side=Left
  wires:
  Constant1/1 -> Add/2
  Rate Transition1/1 -> PWM Generator/1
  m/1 -> Add/1
  Gain1/1 -> Rate Transition1/1
  PWM Generator/1 -> Gain/1
  Add/1 -> Gain1/1
  Protection/1(G1) -> Simulink-PS Converter1/1
  Protection/2(G2) -> Simulink-PS Converter/1
  Gain/1 -> Protection/1(G)
  TripSig/1 -> Protection/2(TripSig)
  connections:
  Four-Pulse Gate Multiplexer1/LConn3 -- Four-Pulse Gate Multiplexer1/LConn2 -- Simulink-PS Converter/RConn1
  P/RConn1 -- Four-Quadrant Chopper1/RConn1
  Four-Pulse Gate Multiplexer1/LConn1 -- Four-Pulse Gate Multiplexer1/LConn4 -- Simulink-PS Converter1/RConn1
  Four-Quadrant Chopper1/RConn2 -- N/RConn1
  -/RConn1 -- Four-Quadrant Chopper1/LConn3
  Four-Quadrant Chopper1/LConn1 -- Four-Pulse Gate Multiplexer1/RConn1
  +/RConn1 -- Four-Quadrant Chopper1/LConn2

== system EE684_Project/PV Control/Maximum Power Point/MPPT/Initialize ==
  In : Inport
  Constant : Constant  Value=solarPlant.startMPPTValue
  Constant2 : Constant
  Integrator : Integrator
  Switch1 : Switch  Criteria=u2 > Threshold  Threshold=solarPlant.startMPPTValue  SaturateOnIntegerOverflow=off  InputSameDT=off
  Switch2 : Switch  Criteria=u2 > Threshold  Threshold=solarPlant.timeMPPT  SaturateOnIntegerOverflow=off  InputSameDT=off
  Out : Outport
  wires:
  Constant/1 -> Switch1/3
  Switch1/1 -> Switch2/1
  In/1 -> Switch1/2, Switch1/1
  Switch2/1 -> Out/1
  Constant2/1 -> Integrator/1
  [Vpvnow] -> Switch2/3
  Integrator/1 -> Switch2/2

== system EE684_Project/PV Control/Maximum Power Point/MPPT/MPPT Algorithm ==
  Ipv : Inport
  Vpv : Inport  Port=2
  IncrementalConductance : Subsystem  VariantControl=incrementalConductance
  PerturbationAndObsrvation : Subsystem  VariantControl=perturbationAndObservation
  Vmpp : Outport  VectorParamsAs1DForOutWhenUnconnected=off

== system EE684_Project/PV Control/Maximum Power Point/MPPT Subsystem/Current control ==
  e : Inport
  Integrator : Integrator  InitialCondition=1  LimitOutput=on  UpperSaturationLimit=1  LowerSaturationLimit=-0.5
  Ki : Gain  Gain=1/boostController.mppCurrentZeroTimeConst
  Kp : Gain  Gain=boostController.mppCurrentGain
  Saturation : Saturate  UpperLimit=1  LowerLimit=-0.3
  Sum7 : Sum  Inputs=|++
  u : Outport  VectorParamsAs1DForOutWhenUnconnected=off
  wires:
  Integrator/1 -> Sum7/2
  Saturation/1 -> u/1
  Sum7/1 -> Saturation/1
  e/1 -> Kp/1
  Kp/1 -> Ki/1, Sum7/1
  Ki/1 -> Integrator/1

== system EE684_Project/PV Control/Maximum Power Point/MPPT Subsystem/Voltage control ==
  e : Inport
  1/T : Gain  Gain=1/boostController.mppVoltageZeroTimeConst
  Integrator : Integrator  LimitOutput=on  UpperSaturationLimit=boostController.mppVoltageLoopMax  LowerSaturationLimit=boostController.mppVoltageLoopMin
  Kp : Gain  Gain=boostController.mppVoltageGain
  Saturation : Saturate  UpperLimit=boostController.mppVoltageLoopMax  LowerLimit=boostController.mppVoltageLoopMin
  Sum7 : Sum  Inputs=|++
  u : Outport  VectorParamsAs1DForOutWhenUnconnected=off
  wires:
  Integrator/1 -> Sum7/2
  Saturation/1 -> u/1
  Sum7/1 -> Saturation/1
  e/1 -> Kp/1
  Kp/1 -> 1/T/1, Sum7/1
  1/T/1 -> Integrator/1

== system EE684_Project/AC System/Single Phase Inverter/Power Circuit/Average/Map [-1,1] to [0,1] ==
  PS Add : fl_lib/Physical Signals/Functions/PS Add
  PS Constant : fl_lib/Physical Signals/Sources/PS Constant  constant=1
  PS Gain : fl_lib/Physical Signals/Functions/PS Gain  gain=0.5
  u : PMIOPort  Side=Left
  y : PMIOPort  Port=2  Side=Right
  connections:
  PS Constant/RConn1 -- PS Add/LConn1
  PS Gain/RConn1 -- y/RConn1
  PS Add/RConn1 -- PS Gain/LConn1
  u/RConn1 -- PS Add/LConn2

== system EE684_Project/AC System/Single Phase Inverter/Power Circuit/Discrete/Protection ==
  G : Inport
  TripSig : Inport  Port=2
  Constant : Constant  Value=5
  Constant2 : Constant  Value=0
  NOT : Logic  Operator=NOT  IconShape=distinctive  AllPortsSameDT=off  OutDataTypeStr=boolean
  Subtract : Sum  Inputs=-+
  Switch : Switch  Criteria=u2 > Threshold  SaturateOnIntegerOverflow=off  InputSameDT=off
  Switch1 : Switch  Criteria=u2 > Threshold  SaturateOnIntegerOverflow=off  InputSameDT=off
  G1 : Outport  VectorParamsAs1DForOutWhenUnconnected=off
  G2 : Outport  Port=2  VectorParamsAs1DForOutWhenUnconnected=off
  wires:
  Switch1/1 -> G2/1
  NOT/1 -> Switch/2
  Constant2/1 -> Switch/3, Switch1/1
  Constant/1 -> Subtract/2
  Switch/1 -> G1/1
  Subtract/1 -> Switch1/3
  G/1 -> Switch/1, Subtract/1
  TripSig/1 -> Switch1/2, NOT/1

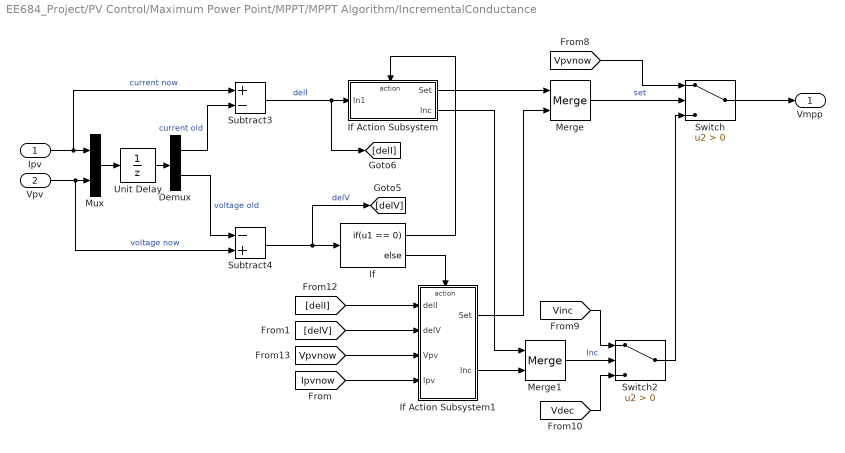
== system EE684_Project/PV Control/Maximum Power Point/MPPT/MPPT Algorithm/IncrementalConductance ==
  Ipv : Inport
  Vpv : Inport  Port=2
  Demux : Demux  Outputs=2
  If : If  IfExpression=u1 == 0
  If Action Subsystem : Subsystem  TreatAsAtomicUnit=on
  If Action Subsystem1 : Subsystem  TreatAsAtomicUnit=on
  Merge : Merge
  Merge1 : Merge
  Mux : Mux  Inputs=2
  Subtract3 : Sum  Inputs=+-
  Subtract4 : Sum  Inputs=-+
  Switch : Switch  Criteria=u2 > Threshold  SaturateOnIntegerOverflow=off  InputSameDT=off
  Switch2 : Switch  Criteria=u2 > Threshold  SaturateOnIntegerOverflow=off  InputSameDT=off
  Unit Delay : UnitDelay  InitialCondition=solarPlant.startMPPTValue  SampleTime=solarPlant.timeMPPT  HasFrameUpgradeWarning=on
  Vmpp : Outport  VectorParamsAs1DForOutWhenUnconnected=off
  wires:
  Merge1/1 -> Switch2/2  "Inc"
  [Vpvnow] -> Switch/1
  If Action Subsystem1/2(Inc) -> Merge1/2
  If Action Subsystem/2(Inc) -> Merge1/1
  If/2 -> If Action Subsystem1/Action
  If Action Subsystem/1(Set) -> Merge/1
  [delV] -> If Action Subsystem1/2(delV)
  [delI] -> If Action Subsystem1/1(delI)
  Merge/1 -> Switch/2  "set"
  If Action Subsystem1/1(Set) -> Merge/2
  If/1 -> If Action Subsystem/Action
  [Vpvnow] -> If Action Subsystem1/3(Vpv)
  Switch2/1 -> Switch/3
  [Ipvnow] -> If Action Subsystem1/4(Ipv)
  Ipv/1 -> Mux/1, Subtract3/1  "current now"
  Unit Delay/1 -> Demux/1
  Mux/1 -> Unit Delay/1
  Vpv/1 -> Subtract4/2, Mux/2  "voltage now"
  Demux/2 -> Subtract4/1  "voltage old"
  Demux/1 -> Subtract3/2  "current old"
  Subtract3/1 -> [delI], If Action Subsystem/1(In1)  "delI"
  Subtract4/1 -> [delV], If/1  "delV"
  Switch/1 -> Vmpp/1
  [Vdec] -> Switch2/3
  [Vinc] -> Switch2/1

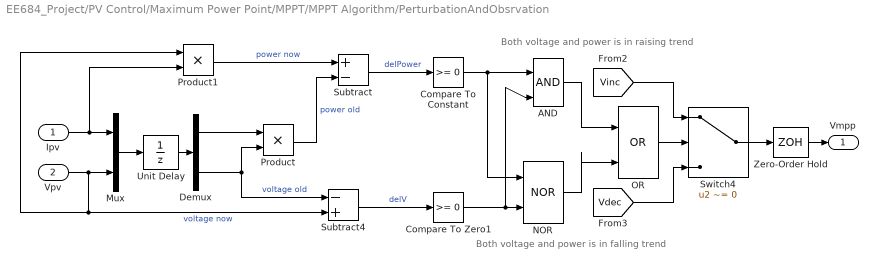
== system EE684_Project/PV Control/Maximum Power Point/MPPT/MPPT Algorithm/PerturbationAndObsrvation ==
  note: Both voltage and power is in falling trend
  note: Both voltage and power is in raising trend
  Ipv : Inport
  Vpv : Inport  Port=2
  AND : Logic  IconShape=distinctive  AllPortsSameDT=off  OutDataTypeStr=boolean
  Compare To Constant : simulink/Logic and Bit Operations/Compare To Constant  relop=>=  const=0  OutDataTypeStr=boolean
  Compare To Zero1 : simulink/Logic and Bit Operations/Compare To Zero  relop=>=  OutDataTypeStr=boolean
  Demux : Demux  Outputs=2
  Mux : Mux  Inputs=2
  NOR : Logic  Operator=NOR  IconShape=distinctive  AllPortsSameDT=off  OutDataTypeStr=boolean
  OR : Logic  Operator=OR  IconShape=distinctive  AllPortsSameDT=off  OutDataTypeStr=boolean
  Product : Product
  Product1 : Product
  Subtract : Sum  Inputs=+-
  Subtract4 : Sum  Inputs=-+
  Switch4 : Switch  Criteria=u2 ~= 0  SaturateOnIntegerOverflow=off  InputSameDT=off
  Unit Delay : UnitDelay  InitialCondition=solarPlant.startMPPTValue  SampleTime=solarPlant.timeMPPT  HasFrameUpgradeWarning=on
  Zero-Order Hold : ZeroOrderHold  SampleTime=solarPlant.timeMPPT
  Vmpp : Outport  VectorParamsAs1DForOutWhenUnconnected=off
  wires:
  NOR/1 -> OR/2
  OR/1 -> Switch4/2
  Compare To Zero1/1 -> AND/2, NOR/2
  AND/1 -> OR/1
  Compare To Constant/1 -> AND/1, NOR/1
  Mux/1 -> Unit Delay/1
  Ipv/1 -> Product1/2, Mux/1
  Demux/1 -> Product/1
  Unit Delay/1 -> Demux/1
  Demux/2 -> Product/2, Subtract4/1  "voltage old"
  Vpv/1 -> Subtract4/2, Product1/1, Mux/2  "voltage now"
  Product1/1 -> Subtract/1  "power now"
  Product/1 -> Subtract/2  "power old"
  Subtract4/1 -> Compare To Zero1/1  "delV"
  Subtract/1 -> Compare To Constant/1  "delPower"
  Switch4/1 -> Zero-Order Hold/1
  [Vdec] -> Switch4/3
  [Vinc] -> Switch4/1
  Zero-Order Hold/1 -> Vmpp/1

== system EE684_Project/PV Control/Maximum Power Point/MPPT/MPPT Algorithm/IncrementalConductance/If Action Subsystem ==
  In1 : Inport
  Action Port : ActionPort  ActionPortLabel=if(u1 == 0)
  Compare To Constant : simulink/Logic and Bit Operations/Compare To Constant  relop===  const=0  OutDataTypeStr=boolean
  Compare To Zero2 : simulink/Logic and Bit Operations/Compare To Zero  relop=>  OutDataTypeStr=boolean
  Set : Outport  VectorParamsAs1DForOutWhenUnconnected=off
  Inc : Outport  Port=2  VectorParamsAs1DForOutWhenUnconnected=off
  wires:
  Compare To Constant/1 -> Set/1  "Yes"
  Compare To Zero2/1 -> Inc/1  "Yes"
  In1/1 -> Compare To Zero2/1, Compare To Constant/1  "delI"

== system EE684_Project/PV Control/Maximum Power Point/MPPT/MPPT Algorithm/IncrementalConductance/If Action Subsystem1 ==
  delI : Inport
  delV : Inport  Port=2
  Vpv : Inport  Port=3
  Ipv : Inport  Port=4
  Action Port : ActionPort  ActionPortLabel=else
  Add : Sum
  Compare To Zero : simulink/Logic and Bit Operations/Compare To Zero  relop===  OutDataTypeStr=boolean
  Compare To Zero1 : simulink/Logic and Bit Operations/Compare To Zero  relop=>  OutDataTypeStr=boolean
  Divide : Product  Inputs=*/
  Product : Product
  Set : Outport  VectorParamsAs1DForOutWhenUnconnected=off
  Inc : Outport  Port=2  VectorParamsAs1DForOutWhenUnconnected=off
  wires:
  delI/1 -> Divide/1
  delV/1 -> Divide/2
  Divide/1 -> Product/1
  Add/1 -> Compare To Zero1/1, Compare To Zero/1
  Compare To Zero/1 -> Set/1  "set"
  Vpv/1 -> Product/2
  Product/1 -> Add/1
  Ipv/1 -> Add/2
  Compare To Zero1/1 -> Inc/1  "Increase"

== stateflow chart EE684_Project/Mode Control ==
  state Mode2_BatCharge_pvMPPT
    entry:
    pvMPPT=1;
    BatCharge=1;
    modeNum=2;
    overload=0;
    exit:
    pvMPPT=0; BatCharge=0;
  state Start_Mode
    entry:
    ShutDown = 0;
    loadShutDown = 1;
    pvMPPT=0;
    VoltageControl=1;
    BatIsolate=1;
    modeNum=0;
    overload=0;
    exit:
    pvMPPT=0;
    BatIsolate=0;
    VoltageControl=0;
    loadShutDown = 0;
  state Mode5_System_ShutDown
    entry:
    PVoff=1; BatIsolate=1;
    ShutDown =1; modeNum=5;
    exit:
    ShutDown =0; PVoff=0;
    BatIsolate=0;
  state Mode1_batIsolated_pvVoltControl
    entry:
    VoltageControl=1; BatIsolate=1;
    modeNum=1;
    exit:
    VoltageControl=0; BatIsolate=0;
  state Mode6_pvMPPT_BatCharge_noload
    entry:
    pvMPPT=1; BatCharge=1;
    loadShutDown=1; modeNum=6;
    overload=1;
    exit:
    loadShutDown=0; pvMPPT=0;
    BatCharge=0;
  state Mode3_BatDischarge_pvMPPT
    entry:
    pvMPPT=1; BatDischarge=1;
    modeNum=3; overload=0;
    exit:
    pvMPPT=0;  BatDischarge=0;
  state Mode4_night_mode
    entry:
    PVoff=1; BatDischarge=1;
    modeNum=4;
    exit:
    PVoff=0; BatDischarge=0;
  Mode2_BatCharge_pvMPPT -> (junction 121) [order 3] : [Irrad<minIrrad && SoC>minSoC]
  Mode2_BatCharge_pvMPPT -> (junction 131) [order 2] : [Vdc < minVdc && SoC>minSoC]
  (junction 121) -> Mode4_night_mode
  (junction 131) -> (junction 154)
  Mode2_BatCharge_pvMPPT -> (junction 117) [order 5] : [Irrad<minIrrad && SoC<minSoC]
  (junction 132) -> Mode2_BatCharge_pvMPPT : [Vdc > maxVdc && Irrad>minIrrad]
  (junction 117) -> Mode5_System_ShutDown
  (junction 155) -> (junction 132)
  (junction 130) -> Mode2_BatCharge_pvMPPT : [(Irrad >minIrrad && overload==0) || ...
      | (overload==1 && rsflag==1)]
  Mode5_System_ShutDown -> (junction 130)
  Start_Mode -> Mode2_BatCharge_pvMPPT [order 1] : [SoC<minSoC]
  (junction 123) -> Mode2_BatCharge_pvMPPT
  Mode6_pvMPPT_BatCharge_noload -> (junction 123) [order 3] : [rsflag ==1 && Irrad > minIrrad  ...
      | && SoC <= minSoC]
  Mode2_BatCharge_pvMPPT -> (junction 125) [order 4]
  (default) -> Start_Mode
  (junction 125) -> Mode6_pvMPPT_BatCharge_noload : [duration(Vdc<minVdc)>olTime ...
      |  && SoC<minSoC]
  Mode2_BatCharge_pvMPPT -> Mode1_batIsolated_pvVoltControl [order 1] : [(SoC>maxSoC) || ...
      | (duration(Vdc>maxVdc)>olTime)]
  Start_Mode -> Mode3_BatDischarge_pvMPPT [order 2] : [SoC>minSoC]
  Mode1_batIsolated_pvVoltControl -> (junction 126)
  Mode6_pvMPPT_BatCharge_noload -> Mode5_System_ShutDown [order 2] : [(SoC<minSoC && ...
      | Irrad<minIrrad)|| ...
      | SoC>maxSoC]
  (junction 126) -> Mode3_BatDischarge_pvMPPT : [Vdc<minVdc]
  (junction 161) -> Mode5_System_ShutDown
  Mode4_night_mode -> Mode5_System_ShutDown [order 2] : [SoC<minSoC]
  Mode6_pvMPPT_BatCharge_noload -> (junction 127) [order 1] : [SoC>minSoC && rsflag==1]
  (junction 127) -> Mode3_BatDischarge_pvMPPT
  (junction 133) -> Mode6_pvMPPT_BatCharge_noload
  Mode3_BatDischarge_pvMPPT -> (junction 133) [order 2] : [(duration(Vdc<minVdc)>olTime || ...
      |  (SoC<minSoC && Vdc<minVdc)) && Irrad>minIrrad]
  Mode3_BatDischarge_pvMPPT -> (junction 161) [order 3] : [(SoC<minSoC && Irrad<minIrrad) || ( Irrad<minIrrad && duration(Vdc<minVdc)>olTime) ]
  Mode3_BatDischarge_pvMPPT -> (junction 155) [order 1]
  Mode4_night_mode -> Mode3_BatDischarge_pvMPPT [order 1] : [Irrad>minIrrad]
  Mode3_BatDischarge_pvMPPT -> Mode4_night_mode [order 4] : [Irrad<minIrrad && SoC>minSoC]
  (junction 154) -> Mode3_BatDischarge_pvMPPT
  data: Irrad input; Vdc input; SoC input; ShutDown output; maxSoC parameter; maxVdc parameter; minIrrad parameter; minSoC parameter; minVdc parameter; loadShutDown output; VoltageControl output; BatCharge output; BatDischarge output; BatIsolate output; PVoff output; pvMPPT output; modeNum output; rsflag input; overload output; olTime parameter
